simulink model "BuckConverterModel"  (R2020a)
settings: Solver=VariableStepAuto  StartTime=0.0  StopTime=0.2  RelTol=1e-3
values from neighbouring files (symbols this model uses):
  C = 3000e-6    (= 0.003)    [parameter.m]
  fsw = 100e3    (= 100000)    [parameter.m]
  L = 500*10^-6    (= 0.0005)    [parameter.m]
  Load = 1    [parameter.m]
libraries: powerlib x11, powerlib_meascontrol x3
settings Model: Creator=ykamatan  LastModifiedBy=ykamatan
settings SolverCC: ZeroCrossAlgorithm=Adaptive
settings DebuggingCC: IgnoredZcDiagnostic=none

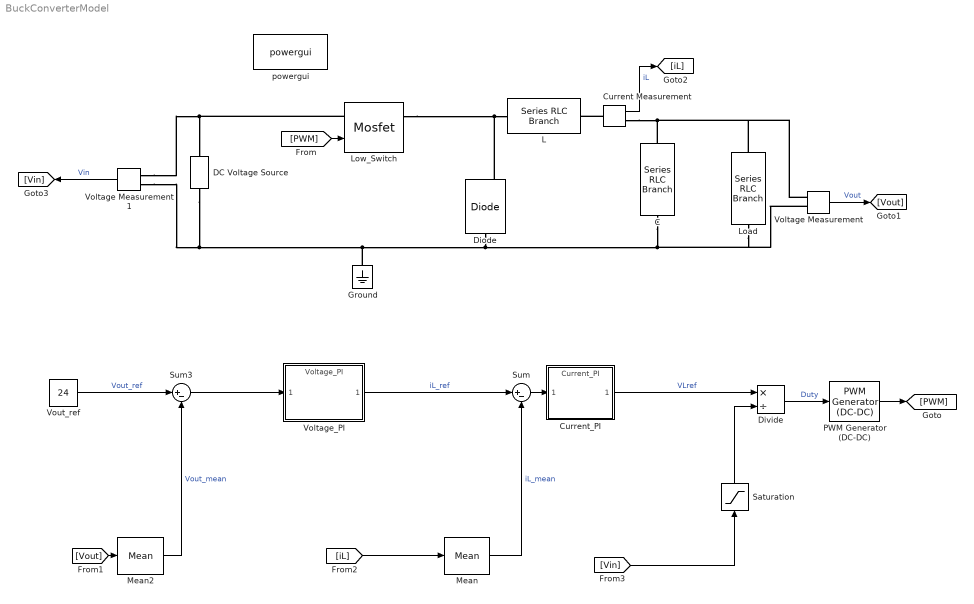
== system BuckConverterModel ==
  C : powerlib/Elements/Series RLC Branch  LConnTagsString=__new0  RConnTagsString=__new0  BranchType=RC  Resistance=10e-3  Inductance=1e-3  SetiL0=off  InitialCurrent=0  Capacitance=C  Setx0=off  InitialVoltage=0  Measurements=None
  Current Measurement : powerlib/Measurements/Current Measurement  PhasorSimulation=off  OutputType=Complex  PSBequivalent=0
  Current_PI : ModelReference  ModelNameDialog=Current_PI  SimulationMode=Normal  ModelReferenceVersion=1.10
  DC Voltage Source : powerlib/Electrical Sources/DC Voltage Source  Amplitude=50  Measurements=None
  Diode : powerlib/Power Electronics/Diode  Ron=0.001  Lon=0  Vf=0  IC=0  UseSnubber=0  Rs=500  Cs=250e-9  Measurements=on
  Divide : Product  Inputs=*/
  Ground : powerlib/Elements/Ground  LConnTagsString=a
  L : powerlib/Elements/Series RLC Branch  LConnTagsString=__new0  RConnTagsString=__new0  BranchType=RL  Resistance=10e-3  Inductance=L  SetiL0=off  InitialCurrent=0  Capacitance=1e-6  Setx0=off  InitialVoltage=0  Measurements=None
  Load : powerlib/Elements/Series RLC Branch  LConnTagsString=__new0  RConnTagsString=__new0  BranchType=R  Resistance=Load  Inductance=1e-3  SetiL0=off  InitialCurrent=0  Capacitance=1e-6  Setx0=off  InitialVoltage=0  Measurements=None
  Low_Switch : powerlib/Power Electronics/Mosfet  Ron=0.001  Lon=0  Rd=0.01  Vfd=0  IC=0  Rs=1e5  Cs=inf  Measurements=on
  Mean : powerlib_meascontrol/Measurements/Mean  Freq=fsw*2  Vinit=0  Ts=1/fsw/2
  Mean2 : powerlib_meascontrol/Measurements/Mean  Freq=fsw*2  Vinit=0  Ts=1/fsw/2
  PWM Generator (DC-DC) : powerlib_meascontrol/Pulse & Signal Generators/PWM Generator (DC-DC)  Fsw=fsw  Ts=0
  Saturation : Saturate  UpperLimit=300  LowerLimit=1
  Sum : Sum  Inputs=|+-
  Sum3 : Sum  Inputs=|+-
  Voltage Measurement : powerlib/Measurements/Voltage Measurement  PhasorSimulation=off  OutputType=Complex  PSBequivalent=0
  Voltage Measurement1 : powerlib/Measurements/Voltage Measurement  PhasorSimulation=off  OutputType=Complex  PSBequivalent=0
  Voltage_PI : ModelReference  ModelNameDialog=Voltage_PI  SimulationMode=Normal  ModelReferenceVersion=1.10
  Vout_ref : Constant  Value=24
  powergui : powerlib/powergui  Priority=1  SimulationMode=Continuous  SampleTime=50e-6  frequency=60  Iterations=50  frequencyindice=0  Pbase=100e6  ErrMax=1e-4  UnitsV=kV  UnitsW=MW  buscounter=0  FunctionMessages=off  echomessages=off  EnableUseOfTLC=off  CurrentSourceSwitches=off  DisableSnubberDevices=off  DisableRonSwitches=off  DisableVfSwitches=off  DisplayEquations=off  AutomaticDiscreteSolvers=off  SolverType=Tustin/Backward Euler (TBE)  Interpol=off  ExternalGateDelay=off  methode=off  Ts=100  x0status=blocks  SPID=on  SwTol=0  HookPort=off  NonlinearTolerance=1e-4  nMaxIteration=100  ContinueOnMaxIteration=off  RestoreLinks=warning  ResistiveCurrentMeasurement=off  Frange=[0:2:500]  Ylog=off  Xlog=on  ShowGrid=off  save=off  variable=ZData  structure=0  ZoomFFT=off  StartTime=0.0  cycles=1  DisplayStyle=1  fundamental=60  FreqAxis=off  MaxFrequency=1000  frequencyindicesteady=1  RmsSteady=1  display=off
  wires:
  PWM Generator (DC-DC)/1 -> [PWM]
  [PWM] -> Low_Switch/1
  Voltage Measurement1/1 -> [Vin]  "Vin"
  Voltage Measurement/1 -> [Vout]  "Vout"
  Current Measurement/1 -> [iL]  "iL"
  [iL] -> Mean/1
  Sum/1 -> Current_PI/1
  Divide/1 -> PWM Generator (DC-DC)/1  "Duty"
  [Vin] -> Saturation/1
  Saturation/1 -> Divide/2
  Vout_ref/1 -> Sum3/1  "Vout_ref"
  Mean/1 -> Sum/2  "iL_mean"
  Current_PI/1 -> Divide/1  "VLref"
  [Vout] -> Mean2/1
  Mean2/1 -> Sum3/2  "Vout_mean"
  Voltage_PI/1 -> Sum/1  "iL_ref"
  Sum3/1 -> Voltage_PI/1
  connections:
  Voltage Measurement1/LConn1 -- DC Voltage Source/RConn1 -- Low_Switch/LConn1
  DC Voltage Source/LConn1 -- Load/RConn1 -- Voltage Measurement/LConn2 -- C/RConn1 -- Diode/LConn1 -- Ground/LConn1 -- Voltage Measurement1/LConn2
  C/LConn1 -- Current Measurement/RConn1 -- Load/LConn1 -- Voltage Measurement/LConn1
  Current Measurement/LConn1 -- L/RConn1
  Low_Switch/RConn1 -- Diode/RConn1 -- L/LConn1
